simulink model "clik_z_inverse"  (R2021b)
settings: Solver=ode1  StartTime=0.0  StopTime=4  FixedStep=0.001  RelTol=1e-3
undefined symbols (not defined in the file or in its folder): DiscIntNeverNeededParam, q0
settings Model: Creator=Xp  LastModifiedBy=rajat
settings SolverCC: AlgebraicLoopSolver=TrustRegion
settings DataIOCC: LimitDataPoints=on  SaveFormat=Array  SignalLoggingSaveFormat=ModelDataLogs  ReturnWorkspaceOutputs=off
settings OptimizationCC: ExpressionDepthLimit=2147483647  InitFltsAndDblsToZero=on  LifeSpan=inf
settings DebuggingCC: SaveWithParameterizedLinksMsg=none  UnderspecifiedInitializationDetection=Classic  MergeDetectMultiDrivingBlocksExec=none  SolverPrmCheckMsg=warning  MultiTaskDSMMsg=warning  MultiTaskCondExecSysMsg=none  FcnCallInpInsideContextMsg=warning  StateNameClashWarn=warning  SFUnexpectedBacktrackingDiag=warning  SFNoUnconditionalDefaultTransitionDiag=warning  SFExecutionAtInitializationDiag=none  SFMachineParentedDataDiag=warning  ArithmeticOperatorsInVariantConditions=warning
settings HardwareCC: ProdBitPerPointer=32  ProdBitPerSizeT=32  ProdBitPerPtrDiffT=32  ProdLargestAtomicFloat=None  ProdIntDivRoundTo=Undefined  ProdEndianess=Unspecified  ProdWordSize=32  ProdHWDeviceType=32-bit Generic
settings ModelReferenceCC: PropagateSignalLabelsOutOfModel=off
settings SFSimCC: CustomCodeUndefinedFunction=UseInterfaceOnly
settings CodeAppCC: StateflowObjectComments=on
settings GRTTargetCC: TargetLangStandard=C89/C90 (ANSI)  CombineOutputUpdateFcns=off  GRTInterface=on
settings ConfigComp: CovMetricSettings=dw  CovSaveCumulativeToWorkspaceVar=on  CovSaveSingleToWorkspaceVar=on

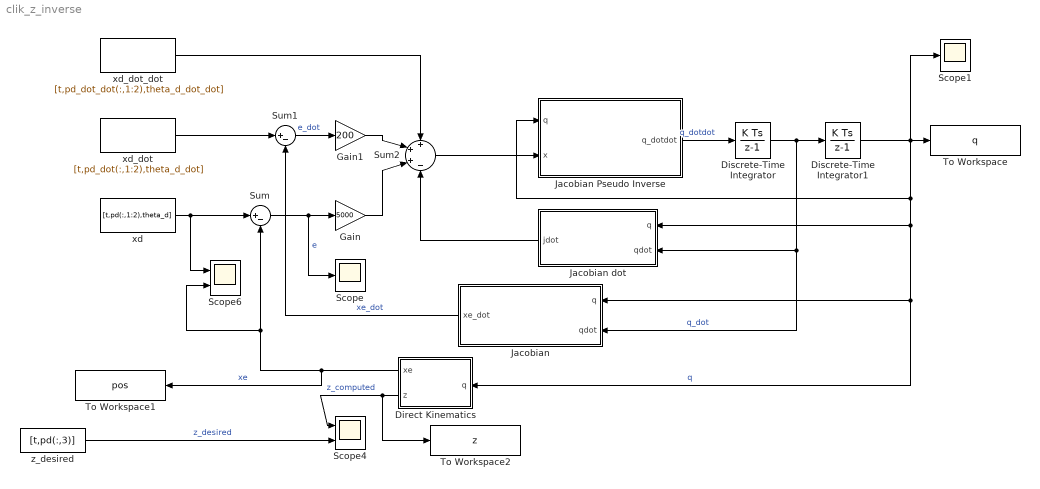
== system clik_z_inverse ==
  Direct Kinematics : MATLAB Function  TreatAsAtomicUnit=on
  Discrete-Time Integrator : DiscreteIntegrator  SampleTime=-1  ICPrevOutput=DiscIntNeverNeededParam  ICPrevScaledInput=DiscIntNeverNeededParam
  Discrete-Time Integrator1 : DiscreteIntegrator  InitialCondition=q0  SampleTime=0.001  LimitOutput=on  UpperSaturationLimit=[pi/2;pi/4;1;2*pi]  LowerSaturationLimit=[-pi/2;-pi/2;0.25;-2*pi]  ICPrevOutput=DiscIntNeverNeededParam  ICPrevScaledInput=DiscIntNeverNeededParam
  Gain : Gain  Gain=5000
  Gain1 : Gain  Gain=200
  "Jacobian " : MATLAB Function  TreatAsAtomicUnit=on
  Jacobian Pseudo Inverse : MATLAB Function  TreatAsAtomicUnit=on
  Jacobian dot : MATLAB Function  TreatAsAtomicUnit=on
  Scope : Scope
  Scope1 : Scope
  Scope4 : Scope  NumInputPorts=2
  Scope6 : Scope  NumInputPorts=2
  Sum : Sum  Inputs=|+-
  Sum1 : Sum  Inputs=|+-
  Sum2 : Sum  Inputs=+++-
  To Workspace : ToWorkspace  VariableName=q  SampleTime=0.001
  To Workspace1 : ToWorkspace  VariableName=pos  SampleTime=0.001
  To Workspace2 : ToWorkspace  VariableName=z  SampleTime=0.001
  xd : FromWorkspace  VariableName=[t,pd(:,1:2),theta_d]  SampleTime=0.001
  xd_dot : FromWorkspace  VariableName=[t,pd_dot(:,1:2),theta_d_dot]  SampleTime=0.001
  xd_dot_dot : FromWorkspace  VariableName=[t,pd_dot_dot(:,1:2),theta_d_dot_dot]
  z_desired : FromWorkspace  VariableName=[t,pd(:,3)]
  wires:
  Direct Kinematics/1(xe) -> To Workspace1/1, Scope6/2, Sum/2  "xe"
  xd/1 -> Scope6/1, Sum/1
  Sum/1 -> Scope/1, Gain/1  "e"
  Sum1/1 -> Gain1/1  "e_dot"
  xd_dot/1 -> Sum1/1
  "Jacobian "/1(xe_dot) -> Sum1/2  "xe_dot"
  xd_dot_dot/1 -> Sum2/1
  Gain1/1 -> Sum2/2
  Gain/1 -> Sum2/3
  Jacobian dot/1(jdot) -> Sum2/4
  Sum2/1 -> Jacobian Pseudo Inverse/2(x)
  Jacobian Pseudo Inverse/1(q_dotdot) -> Discrete-Time Integrator/1  "q_dotdot"
  Discrete-Time Integrator/1 -> "Jacobian "/2(qdot), Jacobian dot/2(qdot), Discrete-Time Integrator1/1  "q_dot"
  Discrete-Time Integrator1/1 -> Jacobian Pseudo Inverse/1(q), Jacobian dot/1(q), Direct Kinematics/1(q), "Jacobian "/1(q), To Workspace/1, Scope1/1  "q"
  Direct Kinematics/2(z) -> To Workspace2/1, Scope4/1  "z_computed"
  z_desired/1 -> Scope4/2  "z_desired"

== matlab function clik_z_inverse/Jacobian  ==
  data: q input; xe_dot output; qdot input
function xe_dot = jacobian(q,qdot)

[~,xe_dot,~]  = jacobian_z_relax(q,qdot,0);

end

== matlab function clik_z_inverse/Direct Kinematics ==
  data: q input; xe output; z output
function [xe,z] = direct_kin(q)
xe = [0 0 0];
[xe,z] = direct_kin(q);
end

== matlab function clik_z_inverse/Jacobian dot ==
  data: q input; jdot output; qdot input
function jdot = jacobian_dot(q,qdot)
jdot = jacobian_dot(q,qdot);
end

== matlab function clik_z_inverse/Jacobian Pseudo Inverse ==
  data: q input; x input; q_dotdot output
function q_dotdot  = z_relax(q,x)
q_dotdot  = [0;0;0;0];
[~,~,q_dotdot]  = jacobian_z_relax(q,0,x);
end
